simulink model "Drone_12"  (R2025b)
settings: Solver=VariableStepAuto  StartTime=0.0  StopTime=10  RelTol=1e-3
values from neighbouring files (symbols this model uses):
  A = d_sys.A    [dobling_algorithm.m]
  B = d_sys.B    [dobling_algorithm.m]
  C = d_sys.C    [dobling_algorithm.m]
  x0 = ones(8,1)    [dobling_algorithm.m]
undefined symbols (not defined in the file or in its folder): D
settings Model: Creator=joanx01  LastModifiedBy=gajic

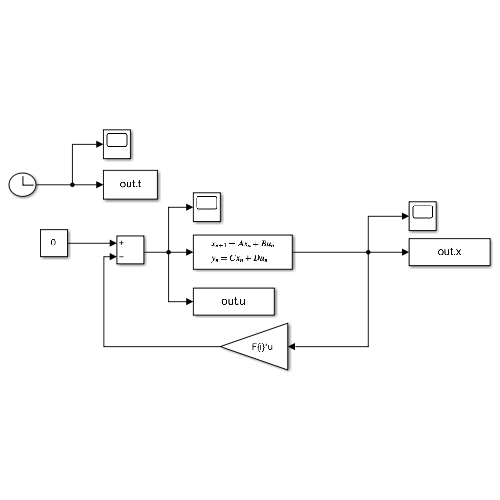
[thumbnail: Simulink's stored preview of the top-level diagram]
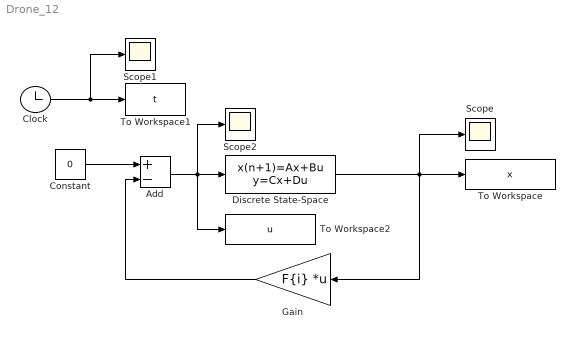
== system Drone_12 ==
  Add : Sum  Inputs=+-
  Clock : Clock
  Constant : Constant  Value=0
  Discrete State-Space : DiscreteStateSpace  A=A  B=B  C=C  D=D  InitialCondition=x0  SampleTime=-1
  Gain : Gain  Gain=F{i}  Multiplication=Matrix(K*u)
  Scope : Scope
      settings: ActiveDisplayYMinimum=-4.5202137866381893  ActiveDisplayYMaximum=1.5031131679991732
  Scope1 : Scope
      settings: ActiveDisplayYMinimum=-1  ActiveDisplayYMaximum=1
  Scope2 : Scope
      settings: ActiveDisplayYMinimum=-1  ActiveDisplayYMaximum=1  DataLoggingVariableName=ScopeData2
  To Workspace : ToWorkspace  VariableName=x  SampleTime=-1
  To Workspace1 : ToWorkspace  VariableName=t  SampleTime=-1
  To Workspace2 : ToWorkspace  VariableName=u  SampleTime=-1
  wires:
  Gain/1 -> Add/2
  Constant/1 -> Add/1
  Discrete State-Space/1 -> Scope/1, To Workspace/1, Gain/1
  Add/1 -> Scope2/1, Discrete State-Space/1, To Workspace2/1
  Clock/1 -> Scope1/1, To Workspace1/1
